simulink model "Es1_sim"  (Simulink 9.2)
settings: Solver=ode45  StartTime=0.0  StopTime=tmax  RelTol=1e-3  EnableMultiTasking=on
values from neighbouring files (symbols this model uses):
  A = [0 1 ... (first row only)    [Es1.m]
  B = [0 1/m]'    [Es1.m]
  C = [1 0]    [Es1.m]
  x0 = [1;1]    [Es1.m]
libraries: simulink x1
settings Model: Creator=professore  LastModifiedBy=utente
settings OptimizationCC: ExpressionDepthLimit=2147483647
settings DebuggingCC: SolverPrmCheckMsg=warning

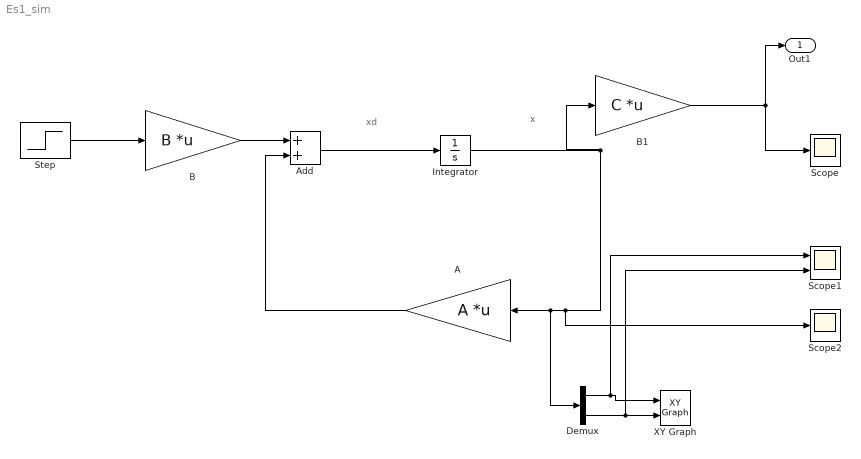
== system Es1_sim ==
  note: xd
  note: x
  A : Gain  Gain=A  Multiplication=Matrix(K*u)
  Add : Sum
  B : Gain  Gain=B  Multiplication=Matrix(K*u)
  B1 : Gain  Gain=C  Multiplication=Matrix(K*u)
  Demux : Demux  Outputs=2
  Integrator : Integrator  InitialCondition=x0
  Scope : Scope
  Scope1 : Scope  NumInputPorts=2
  Scope2 : Scope
  Step : Step  Time=0  After=u  SampleTime=0
  XY Graph : simulink/Sinks/XY Graph  xmin=-5  xmax=5  ymin=-5  ymax=5  st=-1
  Out1 : Outport
  wires:
  Integrator/1 -> B1/1, A/1, Demux/1, Scope2/1
  A/1 -> Add/2
  B/1 -> Add/1
  Add/1 -> Integrator/1
  B1/1 -> Scope/1, Out1/1
  Demux/1 -> XY Graph/1, Scope1/1
  Demux/2 -> XY Graph/2, Scope1/2
  Step/1 -> B/1
